simulink model "Simulacion_de_ecuaciones_diferenciales"  (R2023a)
settings: Solver=VariableStepAuto  StartTime=0.0  StopTime=10.0  RelTol=1e-3
settings Model: Creator=Nacho Andrade  LastModifiedBy=Nacho Andrade

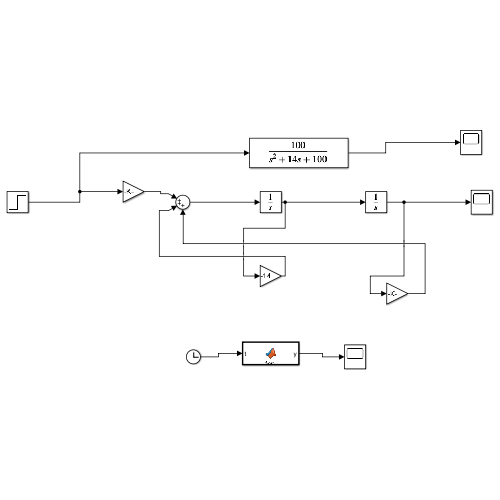
[thumbnail: Simulink's stored preview of the top-level diagram]
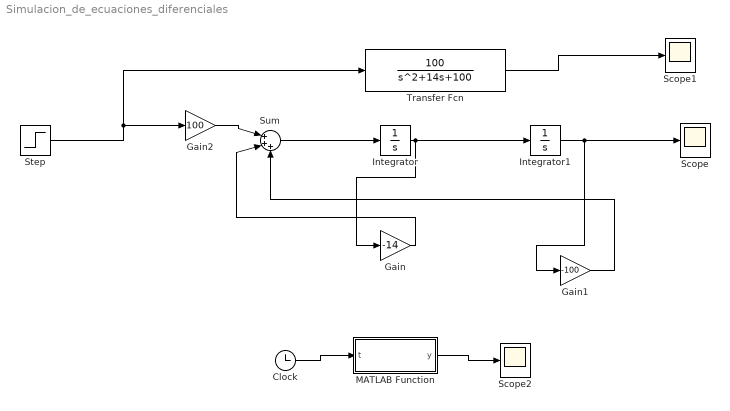
== system Simulacion_de_ecuaciones_diferenciales ==
  Clock : Clock
  Gain : Gain  Gain=-14
  Gain1 : Gain  Gain=-100
  Gain2 : Gain  Gain=100
  Integrator : Integrator
  Integrator1 : Integrator
  MATLAB Function : MATLAB Function  TreatAsAtomicUnit=on
  Scope : Scope
  Scope1 : Scope
  Scope2 : Scope
  Step : Step  Before=1  SampleTime=0
  Sum : Sum  Inputs=|+++
  Transfer Fcn : TransferFcn  Numerator=[100]  Denominator=[1 14 100]
  wires:
  Integrator/1 -> Gain/1, Integrator1/1
  Sum/1 -> Integrator/1
  Step/1 -> Gain2/1, Transfer Fcn/1
  Integrator1/1 -> Scope/1, Gain1/1
  Gain/1 -> Sum/2
  Gain1/1 -> Sum/3
  Transfer Fcn/1 -> Scope1/1
  Clock/1 -> MATLAB Function/1(t)
  MATLAB Function/1(y) -> Scope2/1
  Gain2/1 -> Sum/1

== matlab function Simulacion_de_ecuaciones_diferenciales/MATLAB Function ==
  data: t input; y output
function y = fcn(t)

y = 1/4 - (1)*exp(-3*t) + (3/4)*exp(-4*t);
